simulink model "Pendolo_Inverso"  (R2024a)
settings: Solver=FixedStepAuto  StartTime=0.0  StopTime=10.0  FixedStep=Tc  RelTol=1e-3  EnableMultiTasking=on
values from neighbouring files (symbols this model uses):
  Tc = 0.005    [LoadData.m]
libraries: arduinolib x6, simulink x2, simulink_extras x1
settings Model: ExtModeTrigDuration=2  Creator=josep  LastModifiedBy=josep
settings SolverCC: AutoInsertRateTranBlk=on
settings OptimizationCC: EnhancedBackFolding=on  PassReuseOutputArgsAs=Individual arguments  ZeroExternalMemoryAtStartup=off  ZeroInternalMemoryAtStartup=off  MaxStackSize=64  OptimizeBlockOrder=speed  DifferentSizesBufferReuse=on  OptimizationCustomize=off  EfficientTunableParamExpr=on
settings DebuggingCC: ParameterTunabilityLossMsg=error
settings HardwareCC: ProdBitPerInt=16  ProdBitPerPointer=16  ProdBitPerSizeT=16  ProdBitPerPtrDiffT=16  ProdLargestAtomicFloat=None  ProdWordSize=8  ProdHWDeviceType=Atmel->AVR
settings SFSimCC: MATLABDynamicMemAlloc=off
settings RTWCC: Description=Embedded Coder  SystemTargetFile=ert.tlc  HardwareBoard=Arduino Mega 2560  TemplateMakefile=ert_default_tmf  Toolchain=Arduino AVR  BuildConfiguration=Faster Runs
settings CodeAppCC: ForceParamTrailComments=on  IgnoreCustomStorageClasses=off  OperatorAnnotations=on  SimulinkDataObjDesc=on  SFDataObjDesc=on  InsertBlockDesc=on
settings ERTTargetCC: SupportContinuousTime=on  SupportVariableSizeSignals=on  ExtModeTransport=3  ExtModeStaticAlloc=on  ExtModeAutomaticAllocSize=off  ExtModeStaticAllocSize=2048  ExtModeMexFile=ext_xcp  ExtModeIntrfLevel=Level2 - Open

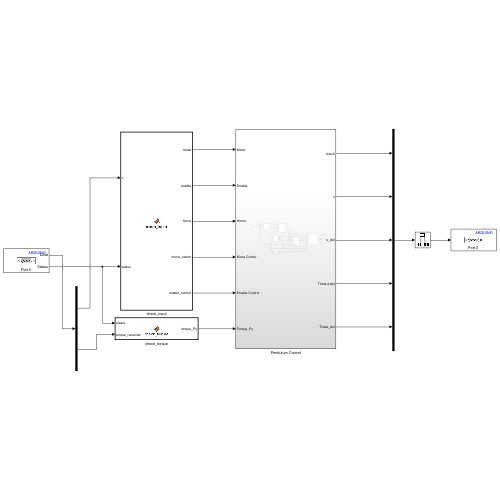
[thumbnail: Simulink's stored preview of the top-level diagram]
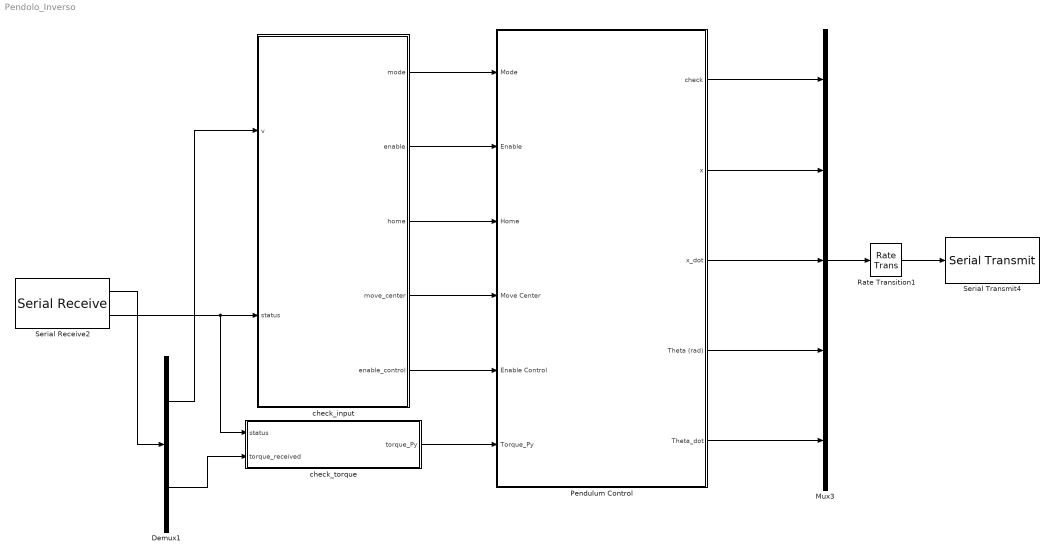
== system Pendolo_Inverso ==
  Demux1 : Demux  Outputs=2
  Mux3 : Mux  Inputs=5
  Pendulum Control : Subsystem
  Rate Transition1 : RateTransition  OutPortSampleTime=0.05
  Serial Receive2 : arduinolib/Serial Receive  isARMArch=off  portNumber=0  DataType=double  DataLengthOption=Length via dialog  MaxDataLength=10  Datalength=2  Header=[]  Terminator=[]  SampleTime=Tc  TimeOut=0  showOutStatus=on  blockPlatform=arduino
  Serial Transmit4 : arduinolib/Serial Transmit  portNumber=0  sendmode=write  sendformat=Decimal  floatprecision=2  header=[]  terminator=[]  blockPlatform=arduino
  check_input : MATLAB Function  TreatAsAtomicUnit=on
  check_torque : MATLAB Function  TreatAsAtomicUnit=on
  wires:
  check_input/2(enable) -> Pendulum Control/2(Enable)
  Serial Receive2/2 -> check_torque/1(status), check_input/2(status)
  check_input/3(home) -> Pendulum Control/3(Home)
  Serial Receive2/1 -> Demux1/1
  Pendulum Control/1(check) -> Mux3/1
  check_input/4(move_center) -> Pendulum Control/4(Move Center)
  Demux1/1 -> check_input/1(v)
  check_input/1(mode) -> Pendulum Control/1(Mode)
  check_torque/1(torque_Py) -> Pendulum Control/6(Torque_Py)
  check_input/5(enable_control) -> Pendulum Control/5(Enable Control)
  Pendulum Control/2(x) -> Mux3/2
  Pendulum Control/3(x_dot) -> Mux3/3
  Pendulum Control/4(Theta (rad)) -> Mux3/4
  Demux1/2 -> check_torque/2(torque_received)
  Pendulum Control/5(Theta_dot) -> Mux3/5
  Mux3/1 -> Rate Transition1/1
  Rate Transition1/1 -> Serial Transmit4/1

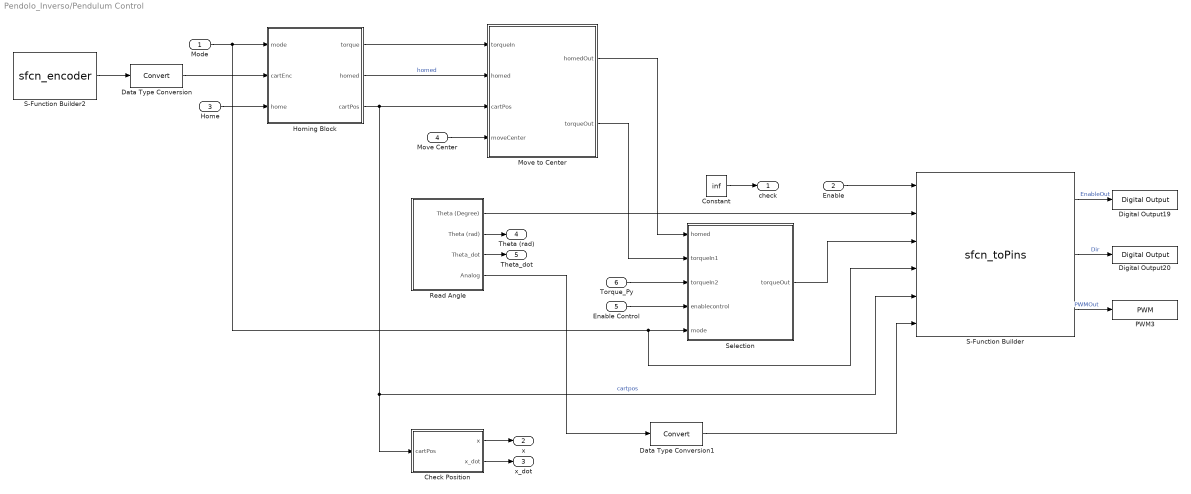
== system Pendolo_Inverso/Pendulum Control ==
  Mode : Inport
  Enable : Inport  Port=2
  Home : Inport  Port=3
  Move Center : Inport  Port=4
  Enable Control : Inport  Port=5
  Torque_Py : Inport  Port=6
  Check Position : Subsystem
  Constant : Constant  Value=inf  OutDataTypeStr=double
  Data Type Conversion : DataTypeConversion  SaturateOnIntegerOverflow=off  RndMeth=Floor
  Data Type Conversion1 : DataTypeConversion  SaturateOnIntegerOverflow=off  RndMeth=Floor
  Digital Output19 : arduinolib/Digital Output  pinNumber=12  Direction=output  blockPlatform=arduino
  Digital Output20 : arduinolib/Digital Output  pinNumber=34  Direction=output  blockPlatform=arduino
  Homing Block : MATLAB Function  TreatAsAtomicUnit=on
  Move to Center : MATLAB Function  TreatAsAtomicUnit=on
  PWM3 : arduinolib/PWM  pinNumber=11  frequencyType=Default  desiredFrequency=490.2  achievableFrequency=490.2
  Read Angle : Subsystem
  S-Function Builder : S-Function  InitFcn=try, set_param(gcb,'FunctionName','sfcn_toPins'), end  FunctionName=sfcn_toPins  SFunctionModules=sfcn_toPins_wrapper.c  SFunctionDeploymentMode=off  EnableBusSupport=off  mask(S-Function Builder){}
      mask help: Simulink:masks:SFunctionBuilder_MD
      mask init:
      | val = [[.9  0.75 0.75 1 1 .9 .9 1]',[1 1 0.75 0.75 .9 .9 1 .9]'];try , sys = get_param(gcb,'SfunBuilderFcnName');if isempty(sys), sys = get_param(gcb,'FunctionName'); end,catch, sys = get_param(gcb,'FunctionName'); end
      settings: CopyFcn=set_param(gcbh,'LinkStatus','none')  PreSaveFcn=try, set_param(gcb,'FunctionName','sfcn_toPins'), end  OpenFcn=sfunctionwizard(gcbh)
      mask Display:
      | plot(val(:,1),val(:,2))
      | disp(sys)
      | port_label('input',1,sprintf('%s', 'Enable'),'interpreter','tex')
      | port_label('input',2,sprintf('%s', 'Analog'),'interpreter','tex')
      | port_label('input',3,sprintf('%s', 'torqueOut'),'interpreter','tex')
      | port_label('input',4,sprintf('%s', 'Mode'),'interpreter','tex')
      | port_label('input',5,sprintf('%s', 'cartPos'),'interpreter','tex')
      | port_label('input',6,sprintf('%s', 'Input'),'interpreter','tex')
      | port_label('output',1,sprintf('%s', 'EnableOut'),'interpreter','tex')
      | port_label('output',2,sprintf('%s', 'Dir'),'interpreter','tex')
      | port_label('output',3,sprintf('%s', 'PWMOut'),'interpreter','tex')
  S-Function Builder2 : S-Function  InitFcn=try, set_param(gcb,'FunctionName','sfcn_encoder'), end  FunctionName=sfcn_encoder  Parameters=uint8(0),uint8(3),uint8(35)  SFunctionModules=sfcn_encoder_wrapper.c  SFunctionDeploymentMode=off  EnableBusSupport=off  mask(S-Function Builder){}
      mask help: Simulink:masks:SFunctionBuilder_MD
      mask init: same as Pendolo_Inverso/Pendulum Control/S-Function Builder
      settings: CopyFcn=set_param(gcbh,'LinkStatus','none')  PreSaveFcn=try, set_param(gcb,'FunctionName','sfcn_encoder'), end  OpenFcn=sfunctionwizard(gcbh)
      mask Display:
      | plot(val(:,1),val(:,2))
      | disp(sys)
      | port_label('output',1,sprintf('%s', 'pos'),'interpreter','tex')
  Selection : MATLAB Function  TreatAsAtomicUnit=on
  check : Outport
  x : Outport  Port=2
  x_dot : Outport  Port=3
  Theta (rad) : Outport  Port=4
  Theta_dot : Outport  Port=5
  wires:
  Enable Control/1 -> Selection/4(enablecontrol)
  S-Function Builder2/1 -> Data Type Conversion/1
  Mode/1 -> S-Function Builder/4, Selection/5(mode), Homing Block/1(mode)
  Enable/1 -> S-Function Builder/1
  Move Center/1 -> Move to Center/4(moveCenter)
  Homing Block/3(cartPos) -> Check Position/1(cartPos), S-Function Builder/5, Move to Center/3(cartPos)  "cartpos"
  Move to Center/1(homedOut) -> Selection/1(homed)
  Data Type Conversion/1 -> Homing Block/2(cartEnc)
  S-Function Builder/3 -> PWM3/1  "PWMOut"
  Constant/1 -> check/1
  Homing Block/2(homed) -> Move to Center/2(homed)  "homed"
  S-Function Builder/2 -> Digital Output20/1  "Dir"
  Home/1 -> Homing Block/3(home)
  Torque_Py/1 -> Selection/3(torqueIn2)
  Data Type Conversion1/1 -> S-Function Builder/6
  Homing Block/1(torque) -> Move to Center/1(torqueIn)
  Move to Center/2(torqueOut) -> Selection/2(torqueIn1)
  S-Function Builder/1 -> Digital Output19/1  "EnableOut"
  Check Position/1(x) -> x/1
  Check Position/2(x_dot) -> x_dot/1
  Read Angle/4(Analog) -> Data Type Conversion1/1
  Read Angle/2(Theta (rad)) -> Theta (rad)/1
  Read Angle/3(Theta_dot) -> Theta_dot/1
  Selection/1(torqueOut) -> S-Function Builder/3
  Read Angle/1(Theta (Degree)) -> S-Function Builder/2

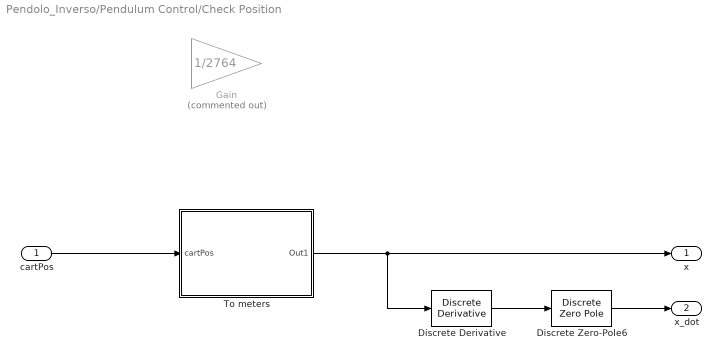
== system Pendolo_Inverso/Pendulum Control/Check Position ==
  cartPos : Inport
  Discrete Zero-Pole6 : DiscreteZeroPole  Zeros=[-e^(-20*Tc)]  Poles=[e^(-20*Tc)]  Gain=20*Tc/2  SampleTime=-1
  Discrete Derivative : simulink/Discrete/Discrete Derivative  gainval=1  ICPrevScaledInput=0.0  OutMin=[]  OutMax=[]  OutDataType=fixdt(1, 16)  OutScaling=2^-10  DoSatur=off
  Gain : Gain  Commented=on  Gain=1/2764
  To meters : Subsystem
  x : Outport
  x_dot : Outport  Port=2
  wires:
  To meters/1(Out1) -> Discrete Derivative/1, x/1
  Discrete Zero-Pole6/1 -> x_dot/1
  Discrete Derivative/1 -> Discrete Zero-Pole6/1
  cartPos/1 -> To meters/1(cartPos)

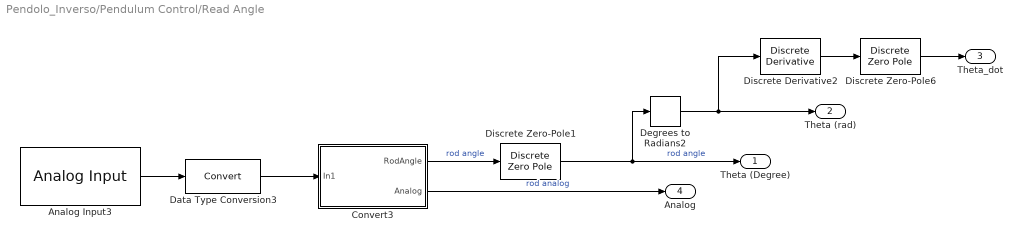
== system Pendolo_Inverso/Pendulum Control/Read Angle ==
  Analog Input3 : arduinolib/Analog Input  pinNumber=5  ReadResultsOnly=off  ConversionTriggerSource=Software  ExternalTriggerType=uint32( 0 )  OutputDataType=uint16  EnableConversionCompleteNotify=off  EnableOuputStatus=off  SampleTime=Tc  blockPlatform=arduino
  Convert3 : Subsystem
  Data Type Conversion3 : DataTypeConversion  SaturateOnIntegerOverflow=off  RndMeth=Floor
  Degrees to Radians2 : simulink_extras/Transformations/Degrees to Radians
  Discrete Zero-Pole1 : DiscreteZeroPole  Zeros=[-e^(-15*Tc)]  Poles=[e^(-15*Tc)]  Gain=15*Tc/2  SampleTime=-1
  Discrete Zero-Pole6 : DiscreteZeroPole  Zeros=[-e^(-20*Tc)]  Poles=[e^(-20*Tc)]  Gain=20*Tc/2  SampleTime=-1
  Discrete Derivative2 : simulink/Discrete/Discrete Derivative  gainval=1  ICPrevScaledInput=0.0  OutMin=[]  OutMax=[]  OutDataType=fixdt(1, 16)  OutScaling=2^-10  DoSatur=off
  Theta (Degree) : Outport
  Theta (rad) : Outport  Port=2
  Theta_dot : Outport  Port=3
  Analog : Outport  Port=4
  wires:
  Discrete Derivative2/1 -> Discrete Zero-Pole6/1
  Discrete Zero-Pole6/1 -> Theta_dot/1
  Degrees to Radians2/1 -> Discrete Derivative2/1, Theta (rad)/1
  Discrete Zero-Pole1/1 -> Degrees to Radians2/1, Theta (Degree)/1  "rod angle"
  Convert3/2(Analog) -> Analog/1  "rod analog"
  Convert3/1(RodAngle) -> Discrete Zero-Pole1/1  "rod angle"
  Data Type Conversion3/1 -> Convert3/1(In1)
  Analog Input3/1 -> Data Type Conversion3/1

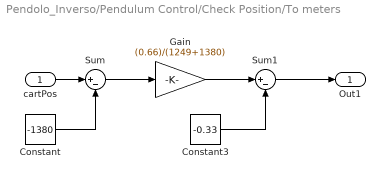
== system Pendolo_Inverso/Pendulum Control/Check Position/To meters ==
  cartPos : Inport
  Constant : Constant  Value=-1380
  Constant3 : Constant  Value=-0.33
  Gain : Gain  Gain=(0.66)/(1249+1380)
  Sum : Sum  Inputs=|+-
  Sum1 : Sum  Inputs=|+-
  Out1 : Outport
  wires:
  cartPos/1 -> Sum/1
  Constant/1 -> Sum/2
  Sum/1 -> Gain/1
  Gain/1 -> Sum1/1
  Sum1/1 -> Out1/1
  Constant3/1 -> Sum1/2

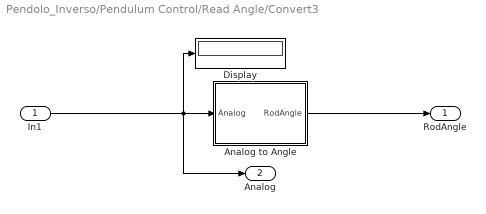
== system Pendolo_Inverso/Pendulum Control/Read Angle/Convert3 ==
  In1 : Inport
  Analog to Angle : Subsystem
  Display : Display
  RodAngle : Outport
  Analog : Outport  Port=2
  wires:
  In1/1 -> Analog/1, Display/1, Analog to Angle/1(Analog)
  Analog to Angle/1(RodAngle) -> RodAngle/1

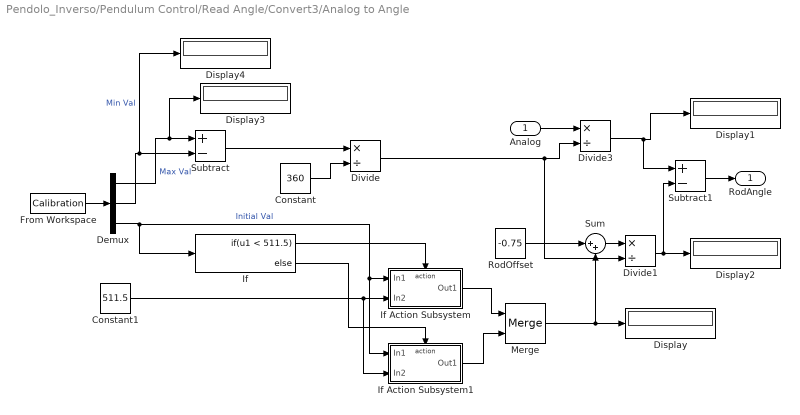
== system Pendolo_Inverso/Pendulum Control/Read Angle/Convert3/Analog to Angle ==
  Analog : Inport
  Constant : Constant  Value=360
  Constant1 : Constant  Value=511.5
  Demux : Demux  Outputs=3
  Display{,1..4} (5 alike) : Display
  Divide : Product  Inputs=*/
  Divide1 : Product  Inputs=*/
  Divide3 : Product  Inputs=*/
  From Workspace : FromWorkspace  VariableName=Calibration
  If : If  IfExpression=u1 < 511.5
  If Action Subsystem : Subsystem  TreatAsAtomicUnit=on
  If Action Subsystem1 : Subsystem  TreatAsAtomicUnit=on
  Merge : Merge
  RodOffset : Constant  Value=-0.75
  Subtract : Sum  Inputs=+-
  Subtract1 : Sum  Inputs=+-
  Sum : Sum  Inputs=|++
  RodAngle : Outport
  wires:
  Demux/3 -> If/1, If Action Subsystem1/1(In1), If Action Subsystem/1(In1)  "Initial Val"
  Constant1/1 -> If Action Subsystem1/2(In2), If Action Subsystem/2(In2)
  If/1 -> If Action Subsystem/Action
  If/2 -> If Action Subsystem1/Action
  If Action Subsystem1/1(Out1) -> Merge/2
  If Action Subsystem/1(Out1) -> Merge/1
  Merge/1 -> Sum/2, Display/1
  Demux/1 -> Display3/1, Subtract/1  "Max Val"
  Demux/2 -> Display4/1, Subtract/2  "Min Val"
  Constant/1 -> Divide/2
  Subtract/1 -> Divide/1
  Divide/1 -> Divide1/2, Divide3/2
  Analog/1 -> Divide3/1
  Divide1/1 -> Display2/1, Subtract1/2
  Divide3/1 -> Display1/1, Subtract1/1
  Subtract1/1 -> RodAngle/1
  RodOffset/1 -> Sum/1
  Sum/1 -> Divide1/1
  From Workspace/1 -> Demux/1

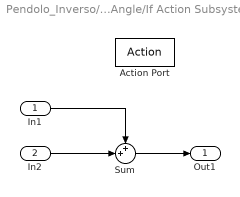
== system Pendolo_Inverso/Pendulum Control/Read Angle/Convert3/Analog to Angle/If Action Subsystem ==
  In1 : Inport
  In2 : Inport  Port=2
  Action Port : ActionPort  ActionPortLabel=if(u1 < 511.5)
  Sum : Sum  Inputs=++|
  Out1 : Outport  VectorParamsAs1DForOutWhenUnconnected=off
  wires:
  In1/1 -> Sum/1
  In2/1 -> Sum/2
  Sum/1 -> Out1/1

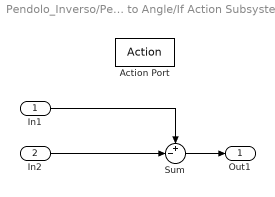
== system Pendolo_Inverso/Pendulum Control/Read Angle/Convert3/Analog to Angle/If Action Subsystem1 ==
  In1 : Inport
  In2 : Inport  Port=2
  Action Port : ActionPort  ActionPortLabel=else
  Sum : Sum  Inputs=+-|
  Out1 : Outport  VectorParamsAs1DForOutWhenUnconnected=off
  wires:
  In1/1 -> Sum/1
  In2/1 -> Sum/2
  Sum/1 -> Out1/1

== matlab function Pendolo_Inverso/check_torque ==
  data: status input; torque_received input; torque_Py output
function torque_Py = check_torque(status, torque_received)

persistent state
persistent torque_value

if(isempty(state))
    state = 1;
    torque_value = 0;
end

if(status == 1)
    torque_value = torque_received;
end

torque_Py = torque_value;

== matlab function Pendolo_Inverso/check_input ==
  data: v input; mode output; enable output; home output; move_center output; enable_control output; status input
function [mode, enable, home, move_center, enable_control] = check_input(v, status)

persistent mode_value
persistent enable_value
persistent home_value
persistent move_center_value
persistent enable_control_value
persistent state

if(isempty(state))
    mode_value = 0;
    enable_value = 0;
    home_value = 0;
    move_center_value = 0;
    enable_control_value = 0;
    state = 0;
end

u = int8(v);
if (status == 1)
    if (u == 1)
        enable_value = mod(enable_value + 1, 2);
    elseif(u == 2)
        home_value = mod(home_value + 1, 2);
    elseif(u == 3)
        move_center_value = mod(move_center_value + 1, 2);
    elseif (u == 4)
        mode_value = mod(mode_value + 1, 2);
    elseif (u == 5)
        enable_control_value = mod(enable_control_value + 1, 2);
    end
end

mode = mode_value;
enable = enable_value;
home = home_value;
move_center = move_center_value;
enable_control = enable_control_value;

== matlab function Pendolo_Inverso/Pendulum Control/Homing Block ==
  settings: updateMethod=DISCRETE
  data: torque output; mode input; cartEnc input; home input; homed output; cartPos output
function [torque,homed,cartPos]=fcn(mode,cartEnc,home)
persistent torqueval
persistent state
persistent precartEnc
persistent homeval
persistent counter
persistent i
persistent precart
persistent prepos
persistent precartArray

% La prima volta isempty(state)==true, quindi inizializza tutte le variabili%
if isempty(state)
    torqueval=0;
    state=0;
    precartEnc=0;
    precartArray=[0 0 0 0 0 0 0 0 0 0];
    homeval=0;
    counter=0;
    i=0;
    precart=0;
    prepos=0;
end

% mode==0 è true se e solo se è settato su Initialize!!!
if (mode==0)

    
    if (homeval==0) % homeval è la variabile homed (homeval==0 : il cart NON sta al limite sinistro, homeval==1 : il cart sta al limite sinistro)
        if (home==0)    %(Home:Value settato ad OFF)
            state=0;
            homeval=0;
            counter=0;
            precart=0;
            prepos=0;
            precartArray=[0 0 0 0 0 0 0 0 0 0];
        end

        if (state==0)   
            torqueval=0;
            if (home==1) % (Home:Value settato ad ON)
                state=1;    % State != 0 <--> Centra il cart
            end
        elseif (state==1)
            torqueval=-300; % Settiamo quanto veloce deve andare il motore (essendo negativo vuol dire che il cart andrà a sinistra)
            state=2;
        elseif (state==2) % 1 sec wait and check final cartpos
            if (counter==150)
                if (all(precartArray==cartEnc)) % Se le ultime 10 posizioni del cart nell'utlimo secondo sono uguali a quella attuale vuol dire che ho raggiunto il limite sinistro
                    torqueval=0;    %Fermo il motore
                    homeval=1;  % Variabile homed settata ad 1
                    prepos=cartEnc; %Salvo il valore encoded della posizione attuale
                else
                      i=i+1;
                      precartArray(i)=precart; %Salvo le ultime 10 posizioni del cart
                      if (i==10)
                          i=0;
                      end             
                      precart=cartEnc;
                end
            else
                counter=counter+1;
            end
        end
    else
        if (home==0)
            state=0;
            homeval=0;
            counter=0;
            precartEnc=0;
            prepos=0;
        end
    end
end
homed=homeval;
torque=torqueval;
if (homed==1)   % Se non siamo più in fase di Inizializzazione prepos è costante, ma cartEnc varia in ogni ciclo
    precartEnc=-1382-prepos; % precartEnc : posizione del limite sinistro del pendolo
    cartPos=precartEnc+cartEnc;     % cartPos : posizione attuale del Cart
else
    cartPos=cartEnc;
end
end

== matlab function Pendolo_Inverso/Pendulum Control/Move to Center ==
  data: homedOut output; torqueIn input; torqueOut output; homed input; cartPos input; moveCenter input
function [homedOut, torqueOut] = fcn(torqueIn, homed, cartPos, moveCenter)
%initializing
persistent kp;
persistent set_pos;
if isempty(kp)
    set_pos=0;
    kp=10;
end

if (homed == 1 && moveCenter==1)    % Se il cart è homed e lo voglio centrare
   torqueOut=(kp*(set_pos-cartPos));    % Imposto un valore della torque proporzionale all'errore
   if (abs(set_pos-cartPos)<1)  % Se sono dentro una banda di tolleranza mi fermo
       torqueOut=0;
   end
else
    torqueOut=torqueIn;
end
homedOut=homed;
end

== matlab function Pendolo_Inverso/Pendulum Control/Selection ==
  settings: updateMethod=DISCRETE
  data: homed input; torqueIn1 input; torqueOut output; torqueIn2 input; enablecontrol input; mode input
function torqueOut  =fcn(homed,torqueIn1,torqueIn2,enablecontrol,mode)
persistent torqueval

if isempty(torqueval)
    torqueval=0;
end

if (mode==0)    % Se è settato su Inizialize
    torqueval=torqueIn1;    % Seguo la torque dettata dal blocco Move To Center
end
if (mode==1)    % Se è settato su Pendulum Control...
    if (homed==1)   %... ed il cart è homed
        if (enablecontrol==1)   % Se Enable Control:Value è settato ad ON
            torqueval=torqueIn2;    % Seguo la torque dettata dal blocco Pendulum Control
        else
            torqueval=0;
        end
    end
end

torqueOut=torqueval;
end
